simulink library "Monika"  (R2025b)
settings: Solver=VariableStepAuto  StartTime=0.0  StopTime=10.0  RelTol=1e-3
undefined symbols (not defined in the file): DiscIntNeverNeededParam, RSN, T_clk, T_maxpoints_maximums
libraries: dspfdesign x3, simulink x3, dspspect3 x1, commsynccomp2 x1
settings Model: Creator=maxim  LastModifiedBy=maxim
settings OptimizationCC: ReuseModelBlockBuffer=off
settings RTWCC: GPUComputeCapability=3.5

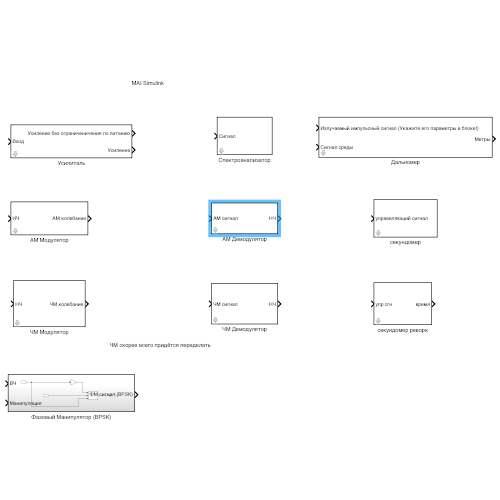
[thumbnail: Simulink's stored preview of the top-level diagram]
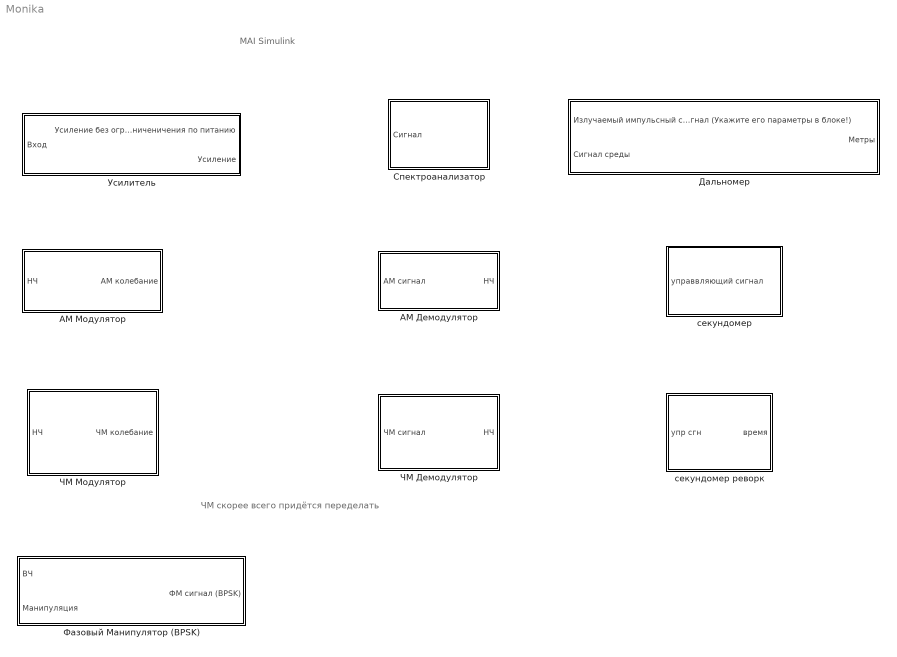
== system Monika ==
  note: MAI Simulink
  note: ЧМ скорее всего придётся переделать
  АМ Демодулятор : Subsystem  mask(АМ Детектор){AD_HF=228, AD_PassbandEdge=10, AD_Order=2}
      mask prompts: AD_HF "Опорная частота (rad/sec)"; AD_PassbandEdge "Верхняя частота пропускания (rad/sec)"; AD_Order "Порядок ФНЧ"
      mask help: Принимает на вход АМ сигнал, из которого "получает" закон модуляции, то есть модулирующий сигнал. В параметрах укажите частоту опорного сигнала (ВЧ), верхнюю частоту пропускания ФНЧ (≈+ 2 rad/sec от НЧ) и его порядок.
      mask Help:
      | Если блок работает неверно, попробуйте следующие действия:
      | * Подвигайте верхнюю частоту пропускания ФНЧ
      | * Измените порядок ФНЧ (большие порядки могут негативно сказываться на работе блока)
      | 
      | Если все эти пункты не помогли, попробуйте удалить блок и поставить его заново (ультимативный метод)
      | 
      | Если и он не помог, соберите его из базовых блоков и напишите замечание нам на Github: https://github.com/Maximon0101/Monika_SimulinkLib
  АМ Модулятор : Subsystem  mask(АМ модулятор){AM_A=1, AM_HF=300, AM_m=1, BAM=on}
      mask prompts: AM_A "Амплитуда ВЧ"; AM_HF "Частота ВЧ (rad/sec)"; AM_m "Глубина"; BAM "БАМ"
      mask help: На вход данного блока поступает модулирующий сигнал (НЧ), а внутри вы указываете параметры параметры несущего сигнала (ВЧ), глубину модуляции, а также то, является ли модуляция балансной (БАМ).
      mask Help:
      | Если модуляция проходит неверно, проверьте следующие пункты:
      | * Частота несущего сигнала (ВЧ) должна быть минимум в 2 раза выше частоты модулирующего (НЧ)
      | * Перепроверьте амплитуды несущего сигнала (в параметрах) и модулирующего (например, с помощью блока Scope)
      | * Проверьте состояние чекбокса БАМ. Попробуйте включить и выключить его
      | 
      | Если все эти пункты не помогли, попробуйте удалить блок и поставить его заново (ультимативный метод)
      | 
      | Если и он не помог, соберите его из базовых блоков и напишите замечание нам на Github: https://github.com/Maximon0101/Monika_SimulinkLib
  Дальномер : Subsystem  mask{T=10, PulseWidth=10}
      mask prompts: T "Период (сек)"; PulseWidth "Ширина импульса (% от Т)"
      mask DialogControl ParameterGroupVar Prompt: Настройка антенны
  Спектроанализатор : Subsystem  mask{SPFS=44100, SPBN=1024, SPS=1}
      mask prompts: SPFS "частота дискретизации (Гц)"; SPBN "ширина кадра (только числа кратные 2)"; SPS "чувствительность (Ом)"
      mask help:
      | Простейший спектроанализатор, выводящий спектр мощности (в децибелах).
      | Настройкой частоты дескретизации регулируется также максимально распознаваемая частота.
      | Рекомедуется изменять частоту дескретизации и ширину кадра 1 к 1
      | Имеется настройка чувствительности.
      mask Help: лучше всего использовать установленные параметры частоты дискретизации и ширины кадра
  Усилитель : Subsystem  mask(Усилитель){Gain=1, dBell_G=Разы, RNS=1, dBell_RSN=Разы, PowerLimit=10, fl=10, fh=228}
      mask prompts: Gain "Усиление"; dBell_G "Множитель усиления"; RNS "ОСШ"; dBell_RSN "Множитель ОСШ"; PowerLimit "Ограничение питания (В)"; fl "Нижняя частота пропускания (Гц)"; fh "Верхняя частота пропускания (Гц)"
      mask help: Блок эмитирует реальный усилитель, усиливая входной сигнал и выводя его с помехами с заданым ОСШ. Также усилитель учитывает ограничение питания сети, к которой он подключён.
      mask Help: Как вы сломали усилитель??? Напишите нам на  Github: https://github.com/Maximon0101/Monika_SimulinkLib
  Фазовый Манипулятор (BPSK) : Subsystem
  ЧМ Демодулятор : Subsystem  mask{FD_HF=228, FD_LF=5, FD_Order=8}
      mask prompts: FD_HF "Опорная частота (ВЧ) (rad/sec)"; FD_LF "Частота НЧ (rad/sec)"; FD_Order "Порядок ФНЧ"
  ЧМ Модулятор : Subsystem  mask{FM_A=10, FM_HF=228, FM_m=40}
      mask prompts: FM_A "Амплитуда ВЧ"; FM_HF "Частота ВЧ (Hz)"; FM_m "Индекс модуляции"
  секундомер : Subsystem  mask{T_clk=T_clk, T_maxpoints_maximums=T_maxpoints_maximums}
      mask prompts: T_clk "период тактирующего сигнала"; T_maxpoints_maximums "ожидаемое количество"
      mask help: считает время от подачи управляющего сигнала, до повторной подачи импульсного сигнала. На выход выдаёт матриуцу из всех проделанных измерений.
  секундомер реворк : Subsystem  mask{T_clk=228}
      mask prompts: T_clk "период тактирующего сигнала"
      mask help: считает время от подачи управляющего сигнала, до повторной подачи импульсного сигнала, выдавая на выход значение текущего или последнего измерения

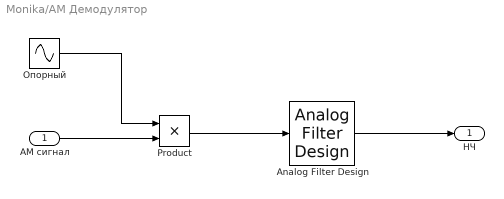
== system Monika/АМ Демодулятор ==
  АМ сигнал : Inport
  Analog Filter Design : dspfdesign/Analog Filter Design  method=Butterworth  filttype=Lowpass  N=AD_Order  Wlo=AD_PassbandEdge  Whi=80  Rp=2  Rs=40
  Product : Product
  Опорный : Sin  Frequency=AD_HF  SampleTime=0
  НЧ : Outport
  wires:
  АМ сигнал/1 -> Product/2
  Опорный/1 -> Product/1
  Analog Filter Design/1 -> НЧ/1
  Product/1 -> Analog Filter Design/1

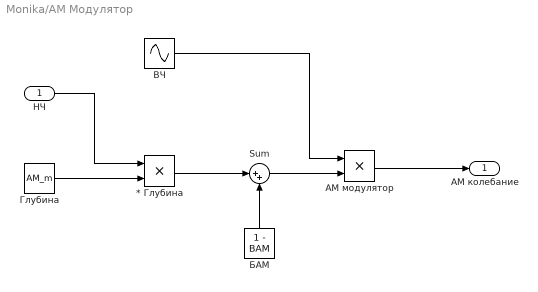
== system Monika/АМ Модулятор ==
  НЧ : Inport
  * Глубина : Product
  Sum : Sum  Inputs=|++
  АМ модулятор : Product
  БАМ : Constant  Value=1 - BAM
  ВЧ : Sin  Amplitude=AM_A  Frequency=AM_HF  SampleTime=0
  Глубина : Constant  Value=AM_m
  АМ колебание : Outport
  wires:
  АМ модулятор/1 -> АМ колебание/1
  НЧ/1 -> * Глубина/1
  Глубина/1 -> * Глубина/2
  * Глубина/1 -> Sum/1
  Sum/1 -> АМ модулятор/2
  БАМ/1 -> Sum/2
  ВЧ/1 -> АМ модулятор/1

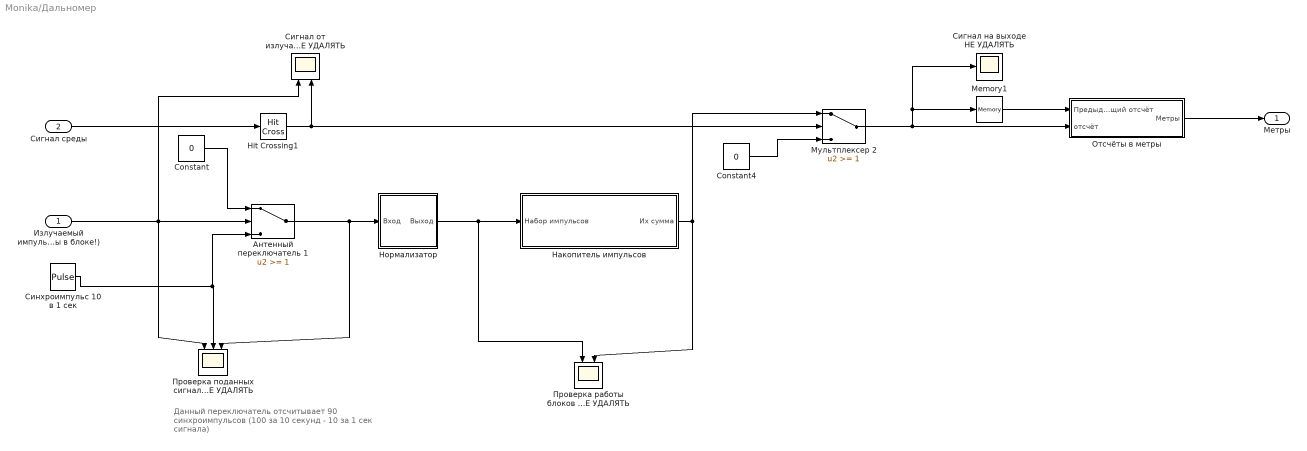
== system Monika/Дальномер ==
  note: Данный переключатель отсчитывает 90 синхроимпульсов (100 за 10 секунд - 10 за 1 сек сигнала)
  Излучаемый импульсный сигнал (Укажите его параметры в блоке!) : Inport
  Сигнал среды : Inport  Port=2
  Constant : Constant  Value=0
  Constant4 : Constant  Value=0
  Hit Crossing1 : HitCross  HitCrossingOffset=0.1  HitCrossingDirection=rising
  Memory1 : Memory
  Антенный переключатель 1 : Switch  Threshold=1  SaturateOnIntegerOverflow=off  InputSameDT=off
  Мультплексер 2 : Switch  Threshold=1  SaturateOnIntegerOverflow=off  InputSameDT=off
  Накопитель импульсов : Subsystem  mask{CountOfPulses=(T * (1 - (PulseWidth*0.01))) * 10}
      mask prompts: CountOfPulses "Количество импульсов"
      mask DialogControl ParameterGroupVar Prompt: Параметры
  Нормализатор : Subsystem
  Отсчёты в метры : Subsystem  mask{CountOfPulses=(T * (1 - (PulseWidth*0.01))) * 10}
      mask prompts: CountOfPulses "Количество импульсов"
      mask DialogControl ParameterGroupVar Prompt: Параметры
  Проверка поданных сигналов НЕ УДАЛЯТЬ : Scope  NumInputPorts=3
      settings: ActiveDisplayYMinimum=-0.24999999999999994  ActiveDisplayYMaximum=2.25  DataLoggingVariableName=ScopeData3
  Проверка работы блоков вокруг НЕ УДАЛЯТЬ : Scope  NumInputPorts=2
      settings: ActiveDisplayYMinimum=-0.12499999999999997  ActiveDisplayYMaximum=1.125
  Сигнал на выходе НЕ УДАЛЯТЬ : Scope
      settings: ActiveDisplayYMinimum=-6.2499999999999982  ActiveDisplayYMaximum=56.25  DataLoggingVariableName=ScopeData2
  Сигнал от излучателя и принятый от цели НЕ УДАЛЯТЬ : Scope  NumInputPorts=2
      settings: ActiveDisplayYMinimum=-0.24999999999999994  ActiveDisplayYMaximum=2.25
  Синхроимпульс 10 в 1 сек : DiscretePulseGenerator  PulseType=Time based  Period=0.1
  Метры : Outport
  wires:
  Накопитель импульсов/1(Их сумма) -> Мультплексер 2/1, Проверка работы блоков вокруг НЕ УДАЛЯТЬ/2
  Нормализатор/1(Выход) -> Проверка работы блоков вокруг НЕ УДАЛЯТЬ/1, Накопитель импульсов/1(Набор импульсов)
  Излучаемый импульсный сигнал (Укажите его параметры в блоке!)/1 -> Антенный переключатель 1/2, Проверка поданных сигналов НЕ УДАЛЯТЬ/1, Сигнал от излучателя и принятый от цели НЕ УДАЛЯТЬ/1
  Hit Crossing1/1 -> Мультплексер 2/2, Сигнал от излучателя и принятый от цели НЕ УДАЛЯТЬ/2
  Constant/1 -> Антенный переключатель 1/1
  Антенный переключатель 1/1 -> Нормализатор/1(Вход), Проверка поданных сигналов НЕ УДАЛЯТЬ/3
  Мультплексер 2/1 -> Отсчёты в метры/2(отсчёт), Сигнал на выходе НЕ УДАЛЯТЬ/1, Memory1/1
  Сигнал среды/1 -> Hit Crossing1/1
  Constant4/1 -> Мультплексер 2/3
  Синхроимпульс 10 в 1 сек/1 -> Проверка поданных сигналов НЕ УДАЛЯТЬ/2, Антенный переключатель 1/3
  Отсчёты в метры/1(Метры) -> Метры/1
  Memory1/1 -> Отсчёты в метры/1(Предыдущий отсчёт)

== system Monika/Спектроанализатор ==
  Сигнал : Inport
  Array Plot1 : ArrayPlot  WindowPosition=[535.000000,197.000000,958.000000,508.000000,]  ScopeFrameLocation=window  SampleIncrement=SPBN/(SPBN*1000)  PlotType=Stairs  AxesScaling=Manual  MaximizeAxes=Off  XLabel=Frequency (kHz)  YLabel=Power (dBm)  YLimits=[-163.8662 33.48879999999999]  ExpandToolstrip=on
  Spectrum Estimator1 : dspspect3/Spectrum Estimator  Method=Filter bank  NumTapsPerBand=SPBN  SpectrumType=Power  FrequencyResolutionMethod=Auto  FilterBankResolutionMethod=Number of frequency bands  RBW=5  WindowLength=1024  FrequencyBandsSource=Specify on dialog  FrequencyBands=SPBN  FFTLengthSource=Auto  FFTLength=1024  InheritSampleRate=on  SampleRate=44100  Window=Hann  SidelobeAttenuation=60  AveragingMethod=Exponential  SpectralAverages=1  ForgettingFactorPort=off  ForgettingFactor=0.9  Overlap=0  ReferenceLoad=SPS  FrequencyRange=One-sided  PowerUnits=dBm  SimulateUsing=Interpreted execution  OutputMaxHoldSpectrum=off  OutputMinHoldSpectrum=off  OutputFrequencyVector=off  OutputRBW=off
  Zero-Order Hold1 : ZeroOrderHold  SampleTime=1/SPFS
  wires:
  Zero-Order Hold1/1 -> Spectrum Estimator1/1
  Spectrum Estimator1/1 -> Array Plot1/1
  Сигнал/1 -> Zero-Order Hold1/1

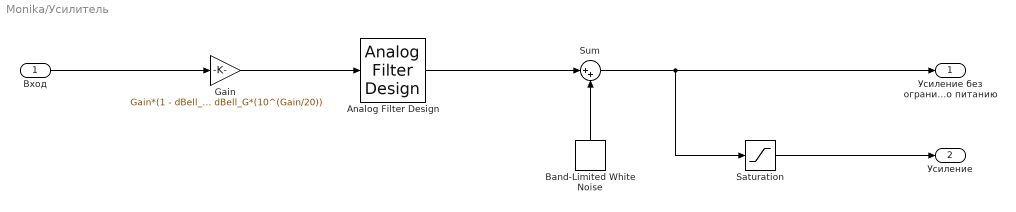
== system Monika/Усилитель ==
  Вход : Inport
  Analog Filter Design : dspfdesign/Analog Filter Design  method=Butterworth  filttype=Bandpass  N=8  Wlo=fl  Whi=fh  Rp=2  Rs=40
  Band-Limited White Noise : simulink/Sources/Band-Limited White Noise  Cov=( Gain*(1 - dBell_G) + dBell_G*(10^(Gain/20)) ) / ( RSN*(1 - dBell_RSN) + dBell_RSN*(10^(RSN/20)) )  Ts=0.00001  seed=[23341]
  Gain : Gain  Gain=Gain*(1 - dBell_G) + dBell_G*(10^(Gain/20))
  Saturation : Saturate  UpperLimit=PowerLimit  LowerLimit=-PowerLimit
  Sum : Sum  Inputs=|++
  Усиление без ограниченичения по питанию : Outport
  Усиление : Outport  Port=2
  wires:
  Saturation/1 -> Усиление/1
  Sum/1 -> Усиление без ограниченичения по питанию/1, Saturation/1
  Вход/1 -> Gain/1
  Band-Limited White Noise/1 -> Sum/2
  Gain/1 -> Analog Filter Design/1
  Analog Filter Design/1 -> Sum/1

== system Monika/Фазовый Манипулятор (BPSK) ==
  ВЧ : Inport
  Манипуляция : Inport  Port=2
  Gain : Gain  Gain=-1
  Switch : Switch  Criteria=u2 > Threshold  SaturateOnIntegerOverflow=off  InputSameDT=off
  ФМ сигнал (BPSK) : Outport
  wires:
  ВЧ/1 -> Gain/1, Switch/3
  Gain/1 -> Switch/1
  Манипуляция/1 -> Switch/2
  Switch/1 -> ФМ сигнал (BPSK)/1

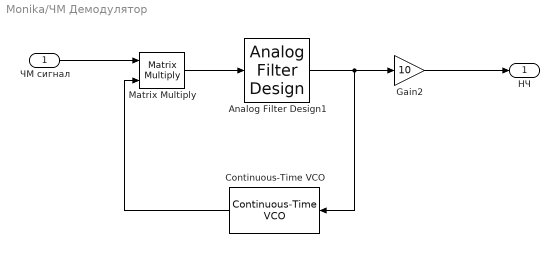
== system Monika/ЧМ Демодулятор ==
  ЧМ сигнал : Inport
  Analog Filter Design1 : dspfdesign/Analog Filter Design  method=Butterworth  filttype=Lowpass  N=FD_Order  Wlo=FD_LF  Whi=80  Rp=2  Rs=40
  Continuous-Time VCO : commsynccomp2/Continuous-Time VCO  Ac=1  Fc=FD_HF  Kc=10/(2*pi)  Ph=pi/2
  Gain2 : Gain  Gain=10
  Matrix Multiply : Product  Multiplication=Matrix(*)
  НЧ : Outport
  wires:
  Analog Filter Design1/1 -> Gain2/1, Continuous-Time VCO/1
  ЧМ сигнал/1 -> Matrix Multiply/1
  Continuous-Time VCO/1 -> Matrix Multiply/2
  Gain2/1 -> НЧ/1
  Matrix Multiply/1 -> Analog Filter Design1/1

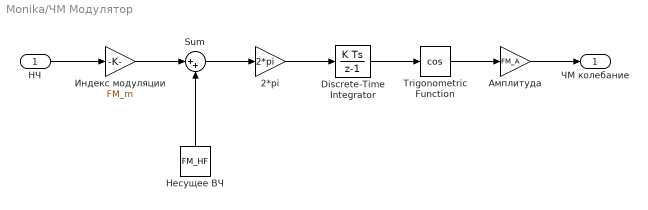
== system Monika/ЧМ Модулятор ==
  НЧ : Inport
  2*pi : Gain  Gain=2*pi
  Discrete-Time Integrator : DiscreteIntegrator  SampleTime=-1  ICPrevOutput=DiscIntNeverNeededParam  ICPrevScaledInput=DiscIntNeverNeededParam
  Sum : Sum  Inputs=|++
  Trigonometric Function : Trigonometry  Operator=cos
  Амплитуда : Gain  Gain=FM_A
  Индекс модуляции : Gain  Gain=FM_m
  Несущее ВЧ : Constant  Value=FM_HF
  ЧМ колебание : Outport
  wires:
  Trigonometric Function/1 -> Амплитуда/1
  Sum/1 -> 2*pi/1
  Индекс модуляции/1 -> Sum/1
  2*pi/1 -> Discrete-Time Integrator/1
  НЧ/1 -> Индекс модуляции/1
  Амплитуда/1 -> ЧМ колебание/1
  Discrete-Time Integrator/1 -> Trigonometric Function/1
  Несущее ВЧ/1 -> Sum/2

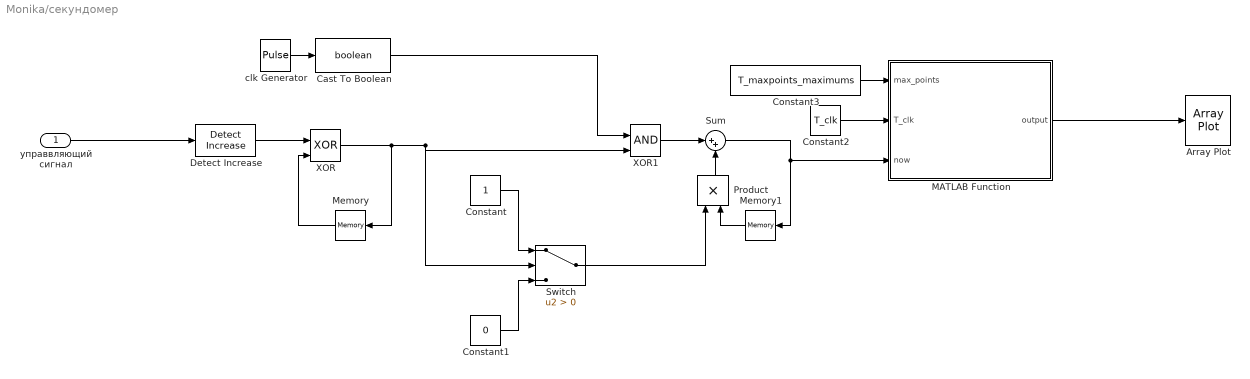
== system Monika/секундомер ==
  управвляющий сигнал : Inport
  Array Plot : ArrayPlot  WindowPosition=[418.000000,174.000000,1338.000000,739.000000,]  ScopeFrameLocation=window  CustomXData=[1,T_maxpoints_maximums]  AxesScaling=Manual  MaximizeAxes=Off  LayoutDimensions=[1 1]  YLabel=Секунды  YLimits=[-1.25 11.25]  ShowLegend=on
  Cast To Boolean : DataTypeConversion  OutDataTypeStr=boolean  SaturateOnIntegerOverflow=off  RndMeth=Floor
  Constant : Constant
  Constant1 : Constant  Value=0
  Constant2 : Constant  Value=T_clk
  Constant3 : Constant  Value=T_maxpoints_maximums
  Detect Increase : simulink/Logic and Bit Operations/Detect Increase  vinit=0.0  OutDataTypeStr=boolean
  MATLAB Function : MATLAB Function  TreatAsAtomicUnit=on
  Memory : Memory  InheritSampleTime=on
  Memory1 : Memory  InheritSampleTime=on
  Product : Product
  Sum : Sum  Inputs=|++
  Switch : Switch  Criteria=u2 > Threshold  SaturateOnIntegerOverflow=off  InputSameDT=off
  XOR : Logic  Operator=XOR  IconShape=distinctive  AllPortsSameDT=off  OutDataTypeStr=boolean
  XOR1 : Logic  IconShape=distinctive  AllPortsSameDT=off  OutDataTypeStr=boolean
  clk Generator : DiscretePulseGenerator  PulseType=Time based  Period=0.1
  wires:
  Product/1 -> Sum/2
  Sum/1 -> Memory1/1, MATLAB Function/3(now)
  MATLAB Function/1(output) -> Array Plot/1
  Constant1/1 -> Switch/3
  XOR/1 -> Memory/1, XOR1/2, Switch/2
  clk Generator/1 -> Cast To Boolean/1
  Memory1/1 -> Product/2
  Cast To Boolean/1 -> XOR1/1
  Constant/1 -> Switch/1
  управвляющий сигнал/1 -> Detect Increase/1
  Switch/1 -> Product/1
  XOR1/1 -> Sum/1
  Memory/1 -> XOR/2
  Detect Increase/1 -> XOR/1
  Constant2/1 -> MATLAB Function/2(T_clk)
  Constant3/1 -> MATLAB Function/1(max_points)

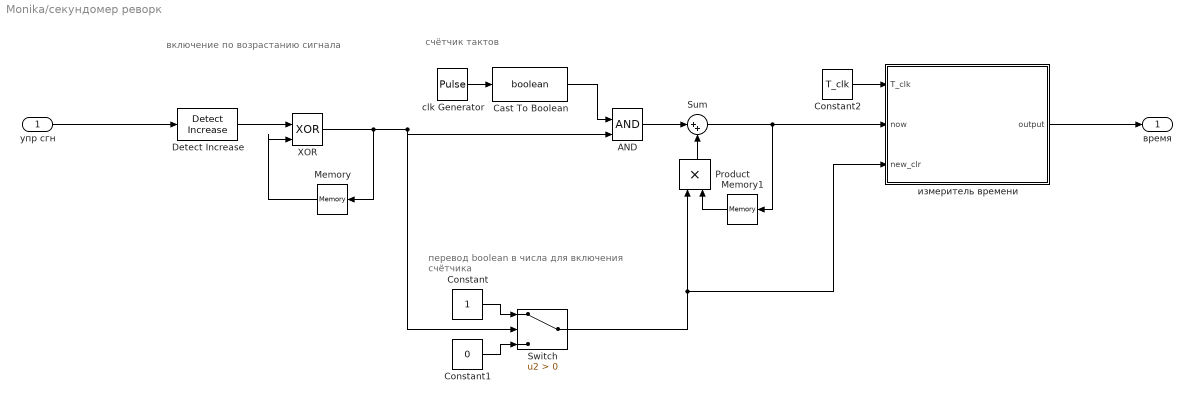
== system Monika/секундомер реворк ==
  note: счётчик тактов
  note: перевод boolean в числа
      | для включения счётчика
  note: включение по возрастанию сигнала
  упр сгн : Inport
  AND : Logic  IconShape=distinctive  AllPortsSameDT=off  OutDataTypeStr=boolean
  Cast To Boolean : DataTypeConversion  OutDataTypeStr=boolean  SaturateOnIntegerOverflow=off  RndMeth=Floor
  Constant : Constant
  Constant1 : Constant  Value=0
  Constant2 : Constant  Value=T_clk
  Detect Increase : simulink/Logic and Bit Operations/Detect Increase  vinit=0.0  OutDataTypeStr=boolean
  Memory : Memory  InheritSampleTime=on
  Memory1 : Memory  InheritSampleTime=on
  Product : Product
  Sum : Sum  Inputs=|++
  Switch : Switch  Criteria=u2 > Threshold  SaturateOnIntegerOverflow=off  InputSameDT=off
  XOR : Logic  Operator=XOR  IconShape=distinctive  AllPortsSameDT=off  OutDataTypeStr=boolean
  clk Generator : DiscretePulseGenerator  PulseType=Time based  Period=T_clk
  измеритель времени : MATLAB Function  TreatAsAtomicUnit=on
  время : Outport
  wires:
  Product/1 -> Sum/2
  Sum/1 -> Memory1/1, измеритель времени/2(now)
  измеритель времени/1(output) -> время/1
  Constant1/1 -> Switch/3
  XOR/1 -> Memory/1, AND/2, Switch/2
  clk Generator/1 -> Cast To Boolean/1
  Memory1/1 -> Product/2
  Cast To Boolean/1 -> AND/1
  Constant/1 -> Switch/1
  упр сгн/1 -> Detect Increase/1
  Switch/1 -> измеритель времени/3(new_clr), Product/1
  AND/1 -> Sum/1
  Memory/1 -> XOR/2
  Constant2/1 -> измеритель времени/1(T_clk)
  Detect Increase/1 -> XOR/1

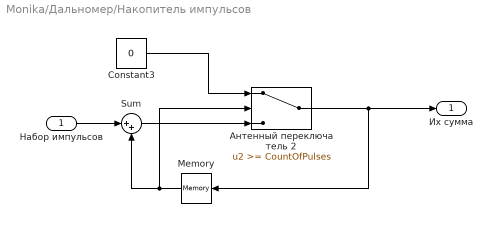
== system Monika/Дальномер/Накопитель импульсов ==
  Набор импульсов : Inport
  Constant3 : Constant  Value=0
  Memory : Memory
  Sum : Sum  Inputs=|++
  Антенный переключатель 2 : Switch  Threshold=CountOfPulses  SaturateOnIntegerOverflow=off  InputSameDT=off
  Их сумма : Outport
  wires:
  Memory/1 -> Антенный переключатель 2/2, Sum/2
  Constant3/1 -> Антенный переключатель 2/1
  Sum/1 -> Антенный переключатель 2/3
  Антенный переключатель 2/1 -> Их сумма/1, Memory/1
  Набор импульсов/1 -> Sum/1

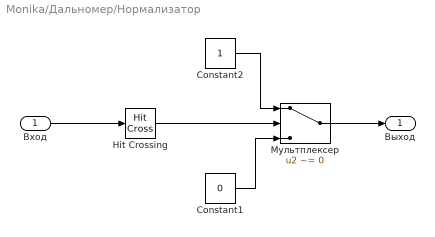
== system Monika/Дальномер/Нормализатор ==
  Вход : Inport
  Constant1 : Constant  Value=0
  Constant2 : Constant
  Hit Crossing : HitCross  HitCrossingOffset=0.1  HitCrossingDirection=rising
  Мультплексер : Switch  Criteria=u2 ~= 0  Threshold=1  SaturateOnIntegerOverflow=off  InputSameDT=off
  Выход : Outport
  wires:
  Constant1/1 -> Мультплексер/3
  Constant2/1 -> Мультплексер/1
  Вход/1 -> Hit Crossing/1
  Hit Crossing/1 -> Мультплексер/2
  Мультплексер/1 -> Выход/1

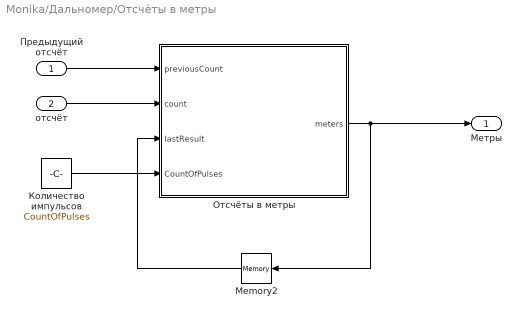
== system Monika/Дальномер/Отсчёты в метры ==
  Предыдущий отсчёт : Inport
  отсчёт : Inport  Port=2
  Memory2 : Memory
  Количество импульсов : Constant  Value=CountOfPulses
  Отсчёты в метры : MATLAB Function  TreatAsAtomicUnit=on
  Метры : Outport
  wires:
  Memory2/1 -> Отсчёты в метры/3(lastResult)
  Количество импульсов/1 -> Отсчёты в метры/4(CountOfPulses)
  Предыдущий отсчёт/1 -> Отсчёты в метры/1(previousCount)
  Отсчёты в метры/1(meters) -> Метры/1, Memory2/1
  отсчёт/1 -> Отсчёты в метры/2(count)

== matlab function Monika/секундомер/MATLAB Function ==
  data: max_points input; T_clk input; now input; output output
function output = maximums(max_points, T_clk, now)
% now - количество тактов
% T_clk - период тактового сигнала в секундах
% output - время в секундах

persistent count;
persistent current_max;
persistent time_buffer;

if isempty(count)
    count = 1;
    current_max = now;
    time_buffer = zeros(max_points, 1);
end

if now > current_max
    current_max = now;
elseif now < current_max
    % Переводим такты в секунды: время = такты * период
    time_buffer(count) = current_max * T_clk;
    count = count + 1;
    current_max = now;
end

output = time_buffer;
end

== matlab function Monika/Дальномер/Отсчёты в метры/Отсчёты в метры ==
  data: previousCount input; meters output; count input; lastResult input; CountOfPulses input
function meters = countsToMeters(previousCount, count, lastResult, CountOfPulses)

if (previousCount > 0 && previousCount < CountOfPulses && count == 0)
    meters = (previousCount * 299792458)/ (10 * 2);
else
    meters = lastResult;
end

== matlab function Monika/секундомер реворк/измеритель времени ==
  data: T_clk input; now input; output output; new_clr input
function output = maximums(T_clk, now, new_clr)

persistent max_in_tacts;
persistent prev_clr;

if isempty(max_in_tacts)
    max_in_tacts = now;
    prev_clr = 0;
end

if now > max_in_tacts
    max_in_tacts = now;
elseif new_clr == 1 && prev_clr == 0
    max_in_tacts = 0;
    prev_clr = 1;
elseif new_clr == 0
    prev_clr = 0;
end

output = max_in_tacts * T_clk;
end
